simulink model "HAE"  (R2018a)
settings: Solver=ode4  StartTime=0  StopTime=2  MaxStep=1e-4  RelTol=1e-3
InitFcn:
  | close
  | clear
  | clc
  | Sc=128
  | f=60;
  | T=1/f;
  | Ts=1/(f*Sc);
  | Vr=6500
  | V_v=[1    0.4    1          0.6       1       0.6       1       0.75   0.95]
  | T_v=[0   20/f  70/f    200/f   300/f     330/f   400/f   500/f  10]
  | S_time=60/f*20.5
  | V_R=3;
  | Tf=3
  | T_lc=3
  | set_param('HAE/EMISOR-RECEPTOR/TCP_IP_RX1/ESCRITURA', 'Value','0')
  | set_param('HAE/EMISOR-RECEPTOR/TCP_IP_RX1/RETARDO', 'Value','0')
  | run script_client_1_inicio2.m
undefined symbols (not defined in the file or in its folder): D11, Delta, DiscIntNeverNeededParam, Int, Ip1
libraries: powerlib x68, simulink x12, powerlib_meascontrol x6, libreria_comunicaciones_cliente2 x2, libreria_medidores2 x1
(part 4 of 5)

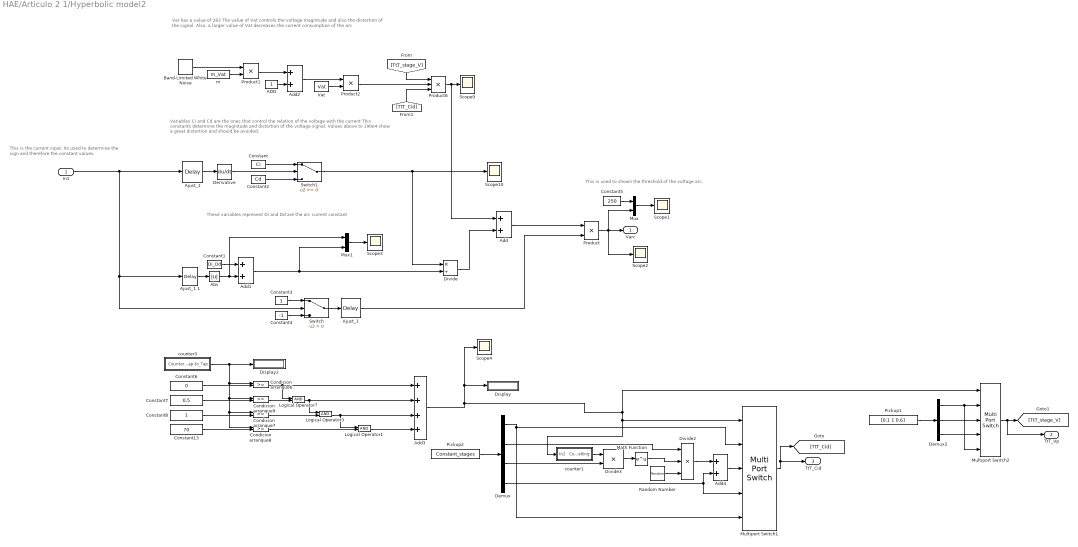
== system HAE/Articulo 2 1/Hyperbolic model2 ==
  note: Vat has a value of 283
      | The value of Vat controls the voltage magnitude and also the distortion of the signal.
      |
      | Also, a larger value of Vat decreases the current consumption of the arc
  note: Variables  Ci and Cd are the ones that control the relation of the voltage with the current
      |
      | This constants determine the magnitude and distortion of the voltage signal.
      |
      | Values above to 190e4 show a great distortion and should be avoided.
  note: These variables represent Di and Dd are the arc current constant
  note: This is used to shown the threshold of the voltage arc.
  note: This is the current input. Its used to determine the sign and therefore the constant values.
  In1 : Inport
  ADD : Constant  SampleTime=Ts
  Abs : Abs
  Add{,1..2,4} (4 alike) : Sum
  Add3 : Sum  Inputs=++++
  Ajust_1 : TransportDelay  DelayTime=1/(1024*60)
  "Ajust_1 " : TransportDelay  DelayTime=1/(1024*60)
  Ajust_1 1 : TransportDelay  DelayTime=1/(1024*60)
  Band-Limited White Noise : simulink/Sources/Band-Limited White Noise  Cov=[0.00005]  Ts=Ts  seed=[500]
  Condicion arranque{6..9} (4 alike) : RelationalOperator  OutDataTypeStr=boolean  RndMeth=Nearest
  Constant : Constant  Value=Ci  SampleTime=Ts
  Constant1 : Constant  Value=Di_Dd  SampleTime=Ts
  Constant13 : Constant  Value=70  VectorParams1D=off  SampleTime=Ts
  Constant2 : Constant  Value=Cd
  Constant3 : Constant
  Constant4 : Constant  Value=-1
  Constant5 : Constant  Value=250
  Constant6 : Constant  Value=0  VectorParams1D=off  SampleTime=Ts
  Constant7 : Constant  Value=0.5  VectorParams1D=off  SampleTime=Ts
  Constant8 : Constant  VectorParams1D=off  SampleTime=Ts
  Demux : Demux
  Demux2 : Demux  Outputs=3
  Derivative : Derivative  CoefficientInTFapproximation=Ts
  Display : Display
  Display2 : Display
  Divide : Product  Inputs=*/
  Divide2 : Product  Inputs=***
  Divide3 : Product  Inputs=**
  Logical Operator1 : Logic  AllPortsSameDT=off  OutDataTypeStr=boolean
  Logical Operator3 : Logic  AllPortsSameDT=off  OutDataTypeStr=boolean
  Logical Operator7 : Logic  AllPortsSameDT=off  OutDataTypeStr=boolean
  Math Function : Math  SaturateOnIntegerOverflow=on
  Multiport Switch1 : MultiPortSwitch  Inputs=4
  Multiport Switch2 : MultiPortSwitch  Inputs=4
  Mux : Mux  Inputs=2
  Mux1 : Mux  Inputs=2
  Pickup1 : Constant  Value=[0.1 1 0.6]
  Pickup2 : Constant  Value=Constant_stages
  Product : Product
  Product1 : Product
  Product2 : Product
  Product6 : Product  Inputs=3
  Random Number : RandomNumber  Mean=2  Variance=0.5  SampleTime=Ts
  Scope{1..4,9..10} (6 alike) : Scope
  Switch : Switch  Criteria=u2 > Threshold  InputSameDT=on
  Switch1 : Switch  InputSameDT=on
  Vat : Constant  Value=Vat  SampleTime=Ts
  counter1 : Subsystem
  counter3 : Subsystem
  "m " : Constant  Value=m_Vat  SampleTime=Ts
  Varc : Outport
  TtT_Vp : Outport  Port=2
  TtT_Cid : Outport  Port=3
  wires:
  Random Number/1 -> Divide2/3
  Add4/1 -> Multiport Switch1/3
  Divide2/1 -> Add4/1
  counter1/1(Counter Melting) -> Divide3/1
  [TtT_Cid] -> Product6/3
  Switch1/1 -> Scope10/1, Divide/1
  Demux2/3 -> Multiport Switch2/4
  Pickup1/1 -> Demux2/1
  Demux2/2 -> Multiport Switch2/3
  Multiport Switch2/1 -> [TtT_stage_V], TtT_Vp/1
  Demux2/1 -> Multiport Switch2/2, Multiport Switch2/5
  Product6/1 -> Scope9/1, Add/1
  Product2/1 -> Product6/2
  [TtT_stage_V] -> Product6/1
  In1/1 -> Ajust_1/1, Ajust_1 1/1, Switch/2
  Add1/1 -> Mux1/2, Divide/2
  Demux/2 -> Divide2/1
  Math Function/1 -> Divide2/2
  Demux/3 -> Divide3/2
  Demux/4 -> Multiport Switch1/4, Add4/2
  Pickup2/1 -> Demux/1
  Divide3/1 -> Math Function/1
  Multiport Switch1/1 -> TtT_Cid/1, [TtT_Cid]
  Demux/1 -> Multiport Switch1/5, Multiport Switch1/2
  Mux1/1 -> Scope3/1
  "Ajust_1 "/1 -> Product/2
  Ajust_1/1 -> Derivative/1
  Derivative/1 -> Switch1/2
  Add2/1 -> Product2/1
  Vat/1 -> Product2/2
  ADD/1 -> Add2/2
  Product1/1 -> Add2/1
  "m "/1 -> Product1/2
  Band-Limited White Noise/1 -> Product1/1
  Abs/1 -> Add1/2, Mux1/1
  Ajust_1 1/1 -> Abs/1
  Constant1/1 -> Add1/1
  Constant5/1 -> Mux/1
  Mux/1 -> Scope1/1
  Constant2/1 -> Switch1/3
  Constant/1 -> Switch1/1
  Product/1 -> Scope2/1, Varc/1, Mux/2
  Switch/1 -> "Ajust_1 "/1
  Constant3/1 -> Switch/1
  Constant4/1 -> Switch/3
  Add/1 -> Product/1
  Divide/1 -> Add/2
  Logical Operator1/1 -> Add3/4
  counter3/1(Counter Tap-to_Tap) -> Condicion arranque9/1, Condicion arranque8/1, Condicion arranque7/1, Condicion arranque6/1, Display2/1
  Condicion arranque7/1 -> Logical Operator3/2
  Logical Operator7/1 -> Add3/2, Logical Operator3/1
  Logical Operator3/1 -> Logical Operator1/1, Add3/3
  Condicion arranque8/1 -> Logical Operator1/2
  Condicion arranque6/1 -> Logical Operator7/1, Add3/1
  Condicion arranque9/1 -> Logical Operator7/2
  Add3/1 -> Multiport Switch2/1, Multiport Switch1/1, counter1/1(In2), Scope4/1, Display/1
  Constant6/1 -> Condicion arranque6/2
  Constant8/1 -> Condicion arranque7/2
  Constant7/1 -> Condicion arranque9/2
  Constant13/1 -> Condicion arranque8/2

== system HAE/Articulo 2 1/counter2 ==
  Add3 : Sum
  Arranq3 : Switch  Threshold=1.5  ZeroCross=off
  Constant1 : Constant  Value=Ts
  Constant3 : Constant  Value=0
  Constant4 : Constant
  Divide : Product  Inputs=**
  Unit Delay1 : UnitDelay  SampleTime=-1
  Unit Delay2 : UnitDelay  SampleTime=-1
  Counter Tap-to_Tap : Outport
  wires:
  Arranq3/1 -> Divide/2
  Add3/1 -> Counter Tap-to_Tap/1, Arranq3/2, Divide/1
  Divide/1 -> Unit Delay1/1
  Constant4/1 -> Arranq3/3
  Constant3/1 -> Arranq3/1
  Unit Delay1/1 -> Add3/2
  Unit Delay2/1 -> Add3/1
  Constant1/1 -> Unit Delay2/1

== system HAE/RB1/RMS1 ==
  In1 : Inport
  Abs : Abs
  Abs1 : Abs
  Abs2 : Abs
  Check zero Crossing : HitCross
  Check zero Crossing1 : HitCross
  Check zero Crossing2 : HitCross
  Constant : Constant  Value=F
  Demux : Demux  Outputs=3
  Discrete Derivative : simulink/Discrete/Discrete Derivative  gainval=1.0  ICPrevScaledInput=0.0  OutMin=[]  OutMax=[]  OutDataType=fixdt(1, 16)  OutScaling=2^-10  DoSatur=off
  Discrete Derivative1 : simulink/Discrete/Discrete Derivative  gainval=1.0  ICPrevScaledInput=0.0  OutMin=[]  OutMax=[]  OutDataType=fixdt(1, 16)  OutScaling=2^-10  DoSatur=off
  Discrete Derivative2 : simulink/Discrete/Discrete Derivative  gainval=1.0  ICPrevScaledInput=0.0  OutMin=[]  OutMax=[]  OutDataType=fixdt(1, 16)  OutScaling=2^-10  DoSatur=off
  Divide : Product  Inputs=/*
  Gain : Gain  Gain=2*pi
  Gain1 : Gain  Gain=1/sqrt(2)
  Hold derivative till next zero crossing : Subsystem  AncestorBlock=|  DialogController=POWERSYS.PowerSysDialog  mask(Discrete Sample & Hold){ic=0, Ts=-1}
      | powerlib_extras/Discrete 
      | Control Blocks/Discrete
      | Sample & Hold
      mask prompts: ic "Initial condition:"; Ts "Sample time:"
      mask help: The output follows input 1 (In) as long as input 2 (S) is TRUE (1) . The output is held when input 2 becomes FALSE (0). The output initial value is specified by the parameter "Initial condition".
      mask init:
      | power_initmask();
      mask Help: This block is part of a subset of blocks in the Extras library that does not have documentation associated with it, other than the block mask description.
      mask Display: disp('S/H')
  Hold derivative till next zero crossing1 : Subsystem  AncestorBlock=|  DialogController=POWERSYS.PowerSysDialog  mask(Discrete Sample & Hold){ic=0, Ts=-1}
      | powerlib_extras/Discrete 
      | Control Blocks/Discrete
      | Sample & Hold
      mask prompts: ic "Initial condition:"; Ts "Sample time:"
      mask help: The output follows input 1 (In) as long as input 2 (S) is TRUE (1) . The output is held when input 2 becomes FALSE (0). The output initial value is specified by the parameter "Initial condition".
      mask init:
      | power_initmask();
      mask Help: This block is part of a subset of blocks in the Extras library that does not have documentation associated with it, other than the block mask description.
      mask Display: disp('S/H')
  Hold derivative till next zero crossing2 : Subsystem  AncestorBlock=|  DialogController=POWERSYS.PowerSysDialog  mask(Discrete Sample & Hold){ic=0, Ts=-1}
      | powerlib_extras/Discrete 
      | Control Blocks/Discrete
      | Sample & Hold
      mask prompts: ic "Initial condition:"; Ts "Sample time:"
      mask help: The output follows input 1 (In) as long as input 2 (S) is TRUE (1) . The output is held when input 2 becomes FALSE (0). The output initial value is specified by the parameter "Initial condition".
      mask init:
      | power_initmask();
      mask Help: This block is part of a subset of blocks in the Extras library that does not have documentation associated with it, other than the block mask description.
      mask Display: disp('S/H')
  Mux : Mux  Inputs=3
  Out1 : Outport
  wires:
  Discrete Derivative/1 -> Hold derivative till next zero crossing/1(In)
  Check zero Crossing/1 -> Hold derivative till next zero crossing/2(S)
  Hold derivative till next zero crossing/1("   ") -> Abs/1
  Constant/1 -> Gain/1
  Gain/1 -> Divide/1
  Abs/1 -> Mux/1
  Demux/1 -> Check zero Crossing/1, Discrete Derivative/1
  Divide/1 -> Gain1/1
  Gain1/1 -> Out1/1
  Hold derivative till next zero crossing1/1("   ") -> Abs1/1
  Check zero Crossing1/1 -> Hold derivative till next zero crossing1/2(S)
  Discrete Derivative1/1 -> Hold derivative till next zero crossing1/1(In)
  Discrete Derivative2/1 -> Hold derivative till next zero crossing2/1(In)
  Check zero Crossing2/1 -> Hold derivative till next zero crossing2/2(S)
  Hold derivative till next zero crossing2/1("   ") -> Abs2/1
  Demux/2 -> Check zero Crossing1/1, Discrete Derivative1/1
  Demux/3 -> Check zero Crossing2/1, Discrete Derivative2/1
  Abs1/1 -> Mux/2
  Mux/1 -> Divide/2
  Abs2/1 -> Mux/3
  In1/1 -> Demux/1

== system HAE/RB1/Timer Proteccion 50 ==
  T.O. : Inport
  Pick-Up : Inport  Port=2
  Entrada : Inport  Port=3
  Arranq3 : Switch  Criteria=u2 ~= 0  Threshold=Ip1
  Arranq6 : Switch  Criteria=u2 ~= 0  Threshold=Ip1  ZeroCross=off
  C14 : Constant  Value=0
  C15 : Constant  Value=1000
  C16 : Constant
  Condicion arranque1 : RelationalOperator  Operator=>  OutDataTypeStr=boolean  RndMeth=Nearest
  Discrete-Time Integrator : DiscreteIntegrator  ExternalReset=falling  SampleTime=-1  ICPrevOutput=DiscIntNeverNeededParam  ICPrevScaledInput=DiscIntNeverNeededParam
  Logical Operator4 : Logic  Operator=NOT  AllPortsSameDT=off  OutDataTypeStr=boolean
  Tiempo Disparo1 : RelationalOperator  OutDataTypeStr=boolean  RndMeth=Nearest
  Trip : Outport
  wires:
  C16/1 -> Arranq6/1
  Arranq6/1 -> Logical Operator4/1, Arranq6/3
  Tiempo Disparo1/1 -> Arranq6/2
  C15/1 -> Arranq3/1
  C14/1 -> Arranq3/3
  Arranq3/1 -> Discrete-Time Integrator/1
  Condicion arranque1/1 -> Arranq3/2, Discrete-Time Integrator/2
  Pick-Up/1 -> Condicion arranque1/2
  Discrete-Time Integrator/1 -> Tiempo Disparo1/1
  Logical Operator4/1 -> Trip/1
  Entrada/1 -> Condicion arranque1/1
  T.O./1 -> Tiempo Disparo1/2

== system HAE/RB1/Timer Proteccion 51 ==
  Entrada : Inport
  Pick-Up : Inport  Port=2
  T.O. : Inport  Port=3
  Arranq3 : Switch  Criteria=u2 ~= 0  Threshold=Ip1
  Arranq6 : Switch  Criteria=u2 ~= 0  Threshold=Ip1  ZeroCross=off
  C14 : Constant  Value=0
  C15 : Constant  Value=1000
  C16 : Constant
  Condicion arranque1 : RelationalOperator  Operator=>  OutDataTypeStr=boolean  RndMeth=Nearest
  Discrete-Time Integrator : DiscreteIntegrator  ExternalReset=falling  SampleTime=-1  ICPrevOutput=DiscIntNeverNeededParam  ICPrevScaledInput=DiscIntNeverNeededParam
  Logical Operator4 : Logic  Operator=NOT  AllPortsSameDT=off  OutDataTypeStr=boolean
  Tiempo Disparo1 : RelationalOperator  OutDataTypeStr=boolean  RndMeth=Nearest
  Trip : Outport
  wires:
  C16/1 -> Arranq6/1
  Arranq6/1 -> Logical Operator4/1, Arranq6/3
  Tiempo Disparo1/1 -> Arranq6/2
  T.O./1 -> Tiempo Disparo1/2
  C15/1 -> Arranq3/1
  C14/1 -> Arranq3/3
  Arranq3/1 -> Discrete-Time Integrator/1
  Condicion arranque1/1 -> Arranq3/2, Discrete-Time Integrator/2
  Pick-Up/1 -> Condicion arranque1/2
  Entrada/1 -> Condicion arranque1/1
  Discrete-Time Integrator/1 -> Tiempo Disparo1/1
  Logical Operator4/1 -> Trip/1

== system HAE/RB4/RMS1 ==
  In1 : Inport
  Abs : Abs
  Abs1 : Abs
  Abs2 : Abs
  Check zero Crossing : HitCross
  Check zero Crossing1 : HitCross
  Check zero Crossing2 : HitCross
  Constant : Constant  Value=F
  Demux : Demux  Outputs=3
  Discrete Derivative : simulink/Discrete/Discrete Derivative  gainval=1.0  ICPrevScaledInput=0.0  OutMin=[]  OutMax=[]  OutDataType=fixdt(1, 16)  OutScaling=2^-10  DoSatur=off
  Discrete Derivative1 : simulink/Discrete/Discrete Derivative  gainval=1.0  ICPrevScaledInput=0.0  OutMin=[]  OutMax=[]  OutDataType=fixdt(1, 16)  OutScaling=2^-10  DoSatur=off
  Discrete Derivative2 : simulink/Discrete/Discrete Derivative  gainval=1.0  ICPrevScaledInput=0.0  OutMin=[]  OutMax=[]  OutDataType=fixdt(1, 16)  OutScaling=2^-10  DoSatur=off
  Divide : Product  Inputs=/*
  Gain : Gain  Gain=2*pi
  Gain1 : Gain  Gain=1/sqrt(2)
  Hold derivative till next zero crossing : Subsystem  AncestorBlock=|  DialogController=POWERSYS.PowerSysDialog  mask(Discrete Sample & Hold){ic=0, Ts=-1}
      | powerlib_extras/Discrete 
      | Control Blocks/Discrete
      | Sample & Hold
      mask prompts: ic "Initial condition:"; Ts "Sample time:"
      mask help: The output follows input 1 (In) as long as input 2 (S) is TRUE (1) . The output is held when input 2 becomes FALSE (0). The output initial value is specified by the parameter "Initial condition".
      mask init:
      | power_initmask();
      mask Help: This block is part of a subset of blocks in the Extras library that does not have documentation associated with it, other than the block mask description.
      mask Display: disp('S/H')
  Hold derivative till next zero crossing1 : Subsystem  AncestorBlock=|  DialogController=POWERSYS.PowerSysDialog  mask(Discrete Sample & Hold){ic=0, Ts=-1}
      | powerlib_extras/Discrete 
      | Control Blocks/Discrete
      | Sample & Hold
      mask prompts: ic "Initial condition:"; Ts "Sample time:"
      mask help: The output follows input 1 (In) as long as input 2 (S) is TRUE (1) . The output is held when input 2 becomes FALSE (0). The output initial value is specified by the parameter "Initial condition".
      mask init:
      | power_initmask();
      mask Help: This block is part of a subset of blocks in the Extras library that does not have documentation associated with it, other than the block mask description.
      mask Display: disp('S/H')
  Hold derivative till next zero crossing2 : Subsystem  AncestorBlock=|  DialogController=POWERSYS.PowerSysDialog  mask(Discrete Sample & Hold){ic=0, Ts=-1}
      | powerlib_extras/Discrete 
      | Control Blocks/Discrete
      | Sample & Hold
      mask prompts: ic "Initial condition:"; Ts "Sample time:"
      mask help: The output follows input 1 (In) as long as input 2 (S) is TRUE (1) . The output is held when input 2 becomes FALSE (0). The output initial value is specified by the parameter "Initial condition".
      mask init:
      | power_initmask();
      mask Help: This block is part of a subset of blocks in the Extras library that does not have documentation associated with it, other than the block mask description.
      mask Display: disp('S/H')
  Mux : Mux  Inputs=3
  Out1 : Outport
  wires:
  In1/1 -> Demux/1
  Abs2/1 -> Mux/3
  Mux/1 -> Divide/2
  Abs1/1 -> Mux/2
  Demux/3 -> Discrete Derivative2/1, Check zero Crossing2/1
  Demux/2 -> Discrete Derivative1/1, Check zero Crossing1/1
  Hold derivative till next zero crossing2/1("   ") -> Abs2/1
  Check zero Crossing2/1 -> Hold derivative till next zero crossing2/2(S)
  Discrete Derivative2/1 -> Hold derivative till next zero crossing2/1(In)
  Discrete Derivative1/1 -> Hold derivative till next zero crossing1/1(In)
  Check zero Crossing1/1 -> Hold derivative till next zero crossing1/2(S)
  Hold derivative till next zero crossing1/1("   ") -> Abs1/1
  Gain1/1 -> Out1/1
  Divide/1 -> Gain1/1
  Demux/1 -> Discrete Derivative/1, Check zero Crossing/1
  Abs/1 -> Mux/1
  Gain/1 -> Divide/1
  Constant/1 -> Gain/1
  Hold derivative till next zero crossing/1("   ") -> Abs/1
  Check zero Crossing/1 -> Hold derivative till next zero crossing/2(S)
  Discrete Derivative/1 -> Hold derivative till next zero crossing/1(In)

== system HAE/RB4/Timer Proteccion 50 ==
  T.O. : Inport
  Pick-Up : Inport  Port=2
  Entrada : Inport  Port=3
  Arranq3 : Switch  Criteria=u2 ~= 0  Threshold=Ip1
  Arranq6 : Switch  Criteria=u2 ~= 0  Threshold=Ip1  ZeroCross=off
  C14 : Constant  Value=0
  C15 : Constant  Value=1000
  C16 : Constant
  Condicion arranque1 : RelationalOperator  Operator=>  OutDataTypeStr=boolean  RndMeth=Nearest
  Discrete-Time Integrator : DiscreteIntegrator  ExternalReset=falling  SampleTime=-1  ICPrevOutput=DiscIntNeverNeededParam  ICPrevScaledInput=DiscIntNeverNeededParam
  Logical Operator4 : Logic  Operator=NOT  AllPortsSameDT=off  OutDataTypeStr=boolean
  Tiempo Disparo1 : RelationalOperator  OutDataTypeStr=boolean  RndMeth=Nearest
  Trip : Outport
  wires:
  T.O./1 -> Tiempo Disparo1/2
  Entrada/1 -> Condicion arranque1/1
  Logical Operator4/1 -> Trip/1
  Discrete-Time Integrator/1 -> Tiempo Disparo1/1
  Pick-Up/1 -> Condicion arranque1/2
  Condicion arranque1/1 -> Discrete-Time Integrator/2, Arranq3/2
  Arranq3/1 -> Discrete-Time Integrator/1
  C14/1 -> Arranq3/3
  C15/1 -> Arranq3/1
  Tiempo Disparo1/1 -> Arranq6/2
  Arranq6/1 -> Arranq6/3, Logical Operator4/1
  C16/1 -> Arranq6/1

== system HAE/RB4/Timer Proteccion 51 ==
  Entrada : Inport
  Pick-Up : Inport  Port=2
  T.O. : Inport  Port=3
  Arranq3 : Switch  Criteria=u2 ~= 0  Threshold=Ip1
  Arranq6 : Switch  Criteria=u2 ~= 0  Threshold=Ip1  ZeroCross=off
  C14 : Constant  Value=0
  C15 : Constant  Value=1000
  C16 : Constant
  Condicion arranque1 : RelationalOperator  Operator=>  OutDataTypeStr=boolean  RndMeth=Nearest
  Discrete-Time Integrator : DiscreteIntegrator  ExternalReset=falling  SampleTime=-1  ICPrevOutput=DiscIntNeverNeededParam  ICPrevScaledInput=DiscIntNeverNeededParam
  Logical Operator4 : Logic  Operator=NOT  AllPortsSameDT=off  OutDataTypeStr=boolean
  Tiempo Disparo1 : RelationalOperator  OutDataTypeStr=boolean  RndMeth=Nearest
  Trip : Outport
  wires:
  Logical Operator4/1 -> Trip/1
  Discrete-Time Integrator/1 -> Tiempo Disparo1/1
  Entrada/1 -> Condicion arranque1/1
  Pick-Up/1 -> Condicion arranque1/2
  Condicion arranque1/1 -> Discrete-Time Integrator/2, Arranq3/2
  Arranq3/1 -> Discrete-Time Integrator/1
  C14/1 -> Arranq3/3
  C15/1 -> Arranq3/1
  T.O./1 -> Tiempo Disparo1/2
  Tiempo Disparo1/1 -> Arranq6/2
  Arranq6/1 -> Arranq6/3, Logical Operator4/1
  C16/1 -> Arranq6/1

== system HAE/RB5/RMS1 ==
  In1 : Inport
  Abs : Abs
  Abs1 : Abs
  Abs2 : Abs
  Check zero Crossing : HitCross
  Check zero Crossing1 : HitCross
  Check zero Crossing2 : HitCross
  Constant : Constant  Value=F
  Demux : Demux  Outputs=3
  Discrete Derivative : simulink/Discrete/Discrete Derivative  gainval=1.0  ICPrevScaledInput=0.0  OutMin=[]  OutMax=[]  OutDataType=fixdt(1, 16)  OutScaling=2^-10  DoSatur=off
  Discrete Derivative1 : simulink/Discrete/Discrete Derivative  gainval=1.0  ICPrevScaledInput=0.0  OutMin=[]  OutMax=[]  OutDataType=fixdt(1, 16)  OutScaling=2^-10  DoSatur=off
  Discrete Derivative2 : simulink/Discrete/Discrete Derivative  gainval=1.0  ICPrevScaledInput=0.0  OutMin=[]  OutMax=[]  OutDataType=fixdt(1, 16)  OutScaling=2^-10  DoSatur=off
  Divide : Product  Inputs=/*
  Gain : Gain  Gain=2*pi
  Gain1 : Gain  Gain=1/sqrt(2)
  Hold derivative till next zero crossing : Subsystem  AncestorBlock=|  DialogController=POWERSYS.PowerSysDialog  mask(Discrete Sample & Hold){ic=0, Ts=-1}
      | powerlib_extras/Discrete 
      | Control Blocks/Discrete
      | Sample & Hold
      mask prompts: ic "Initial condition:"; Ts "Sample time:"
      mask help: The output follows input 1 (In) as long as input 2 (S) is TRUE (1) . The output is held when input 2 becomes FALSE (0). The output initial value is specified by the parameter "Initial condition".
      mask init:
      | power_initmask();
      mask Help: This block is part of a subset of blocks in the Extras library that does not have documentation associated with it, other than the block mask description.
      mask Display: disp('S/H')
  Hold derivative till next zero crossing1 : Subsystem  AncestorBlock=|  DialogController=POWERSYS.PowerSysDialog  mask(Discrete Sample & Hold){ic=0, Ts=-1}
      | powerlib_extras/Discrete 
      | Control Blocks/Discrete
      | Sample & Hold
      mask prompts: ic "Initial condition:"; Ts "Sample time:"
      mask help: The output follows input 1 (In) as long as input 2 (S) is TRUE (1) . The output is held when input 2 becomes FALSE (0). The output initial value is specified by the parameter "Initial condition".
      mask init:
      | power_initmask();
      mask Help: This block is part of a subset of blocks in the Extras library that does not have documentation associated with it, other than the block mask description.
      mask Display: disp('S/H')
  Hold derivative till next zero crossing2 : Subsystem  AncestorBlock=|  DialogController=POWERSYS.PowerSysDialog  mask(Discrete Sample & Hold){ic=0, Ts=-1}
      | powerlib_extras/Discrete 
      | Control Blocks/Discrete
      | Sample & Hold
      mask prompts: ic "Initial condition:"; Ts "Sample time:"
      mask help: The output follows input 1 (In) as long as input 2 (S) is TRUE (1) . The output is held when input 2 becomes FALSE (0). The output initial value is specified by the parameter "Initial condition".
      mask init:
      | power_initmask();
      mask Help: This block is part of a subset of blocks in the Extras library that does not have documentation associated with it, other than the block mask description.
      mask Display: disp('S/H')
  Mux : Mux  Inputs=3
  Out1 : Outport
  wires:
  Discrete Derivative/1 -> Hold derivative till next zero crossing/1(In)
  Check zero Crossing/1 -> Hold derivative till next zero crossing/2(S)
  Hold derivative till next zero crossing/1("   ") -> Abs/1
  Constant/1 -> Gain/1
  Gain/1 -> Divide/1
  Abs/1 -> Mux/1
  Demux/1 -> Check zero Crossing/1, Discrete Derivative/1
  Divide/1 -> Gain1/1
  Gain1/1 -> Out1/1
  Hold derivative till next zero crossing1/1("   ") -> Abs1/1
  Check zero Crossing1/1 -> Hold derivative till next zero crossing1/2(S)
  Discrete Derivative1/1 -> Hold derivative till next zero crossing1/1(In)
  Discrete Derivative2/1 -> Hold derivative till next zero crossing2/1(In)
  Check zero Crossing2/1 -> Hold derivative till next zero crossing2/2(S)
  Hold derivative till next zero crossing2/1("   ") -> Abs2/1
  Demux/2 -> Check zero Crossing1/1, Discrete Derivative1/1
  Demux/3 -> Check zero Crossing2/1, Discrete Derivative2/1
  Abs1/1 -> Mux/2
  Mux/1 -> Divide/2
  Abs2/1 -> Mux/3
  In1/1 -> Demux/1

== system HAE/RB5/Timer Proteccion 50 ==
  T.O. : Inport
  Pick-Up : Inport  Port=2
  Entrada : Inport  Port=3
  Arranq3 : Switch  Criteria=u2 ~= 0  Threshold=Ip1
  Arranq6 : Switch  Criteria=u2 ~= 0  Threshold=Ip1  ZeroCross=off
  C14 : Constant  Value=0
  C15 : Constant  Value=1000
  C16 : Constant
  Condicion arranque1 : RelationalOperator  Operator=>  OutDataTypeStr=boolean  RndMeth=Nearest
  Discrete-Time Integrator : DiscreteIntegrator  ExternalReset=falling  SampleTime=-1  ICPrevOutput=DiscIntNeverNeededParam  ICPrevScaledInput=DiscIntNeverNeededParam
  Logical Operator4 : Logic  Operator=NOT  AllPortsSameDT=off  OutDataTypeStr=boolean
  Tiempo Disparo1 : RelationalOperator  OutDataTypeStr=boolean  RndMeth=Nearest
  Trip : Outport
  wires:
  C16/1 -> Arranq6/1
  Arranq6/1 -> Logical Operator4/1, Arranq6/3
  Tiempo Disparo1/1 -> Arranq6/2
  C15/1 -> Arranq3/1
  C14/1 -> Arranq3/3
  Arranq3/1 -> Discrete-Time Integrator/1
  Condicion arranque1/1 -> Arranq3/2, Discrete-Time Integrator/2
  Pick-Up/1 -> Condicion arranque1/2
  Discrete-Time Integrator/1 -> Tiempo Disparo1/1
  Logical Operator4/1 -> Trip/1
  Entrada/1 -> Condicion arranque1/1
  T.O./1 -> Tiempo Disparo1/2

== system HAE/RB5/Timer Proteccion 51 ==
  Entrada : Inport
  Pick-Up : Inport  Port=2
  T.O. : Inport  Port=3
  Arranq3 : Switch  Criteria=u2 ~= 0  Threshold=Ip1
  Arranq6 : Switch  Criteria=u2 ~= 0  Threshold=Ip1  ZeroCross=off
  C14 : Constant  Value=0
  C15 : Constant  Value=1000
  C16 : Constant
  Condicion arranque1 : RelationalOperator  Operator=>  OutDataTypeStr=boolean  RndMeth=Nearest
  Discrete-Time Integrator : DiscreteIntegrator  ExternalReset=falling  SampleTime=-1  ICPrevOutput=DiscIntNeverNeededParam  ICPrevScaledInput=DiscIntNeverNeededParam
  Logical Operator4 : Logic  Operator=NOT  AllPortsSameDT=off  OutDataTypeStr=boolean
  Tiempo Disparo1 : RelationalOperator  OutDataTypeStr=boolean  RndMeth=Nearest
  Trip : Outport
  wires:
  C16/1 -> Arranq6/1
  Arranq6/1 -> Logical Operator4/1, Arranq6/3
  Tiempo Disparo1/1 -> Arranq6/2
  T.O./1 -> Tiempo Disparo1/2
  C15/1 -> Arranq3/1
  C14/1 -> Arranq3/3
  Arranq3/1 -> Discrete-Time Integrator/1
  Condicion arranque1/1 -> Arranq3/2, Discrete-Time Integrator/2
  Pick-Up/1 -> Condicion arranque1/2
  Entrada/1 -> Condicion arranque1/1
  Discrete-Time Integrator/1 -> Tiempo Disparo1/1
  Logical Operator4/1 -> Trip/1

== system HAE/Subsystem1/RMS ==
  In1 : Inport
  Absolute : MATLABFcn  MATLABFcn=abs
  Check zero Crossing : HitCross
  Constant : Constant  Value=F
  Derivative : Derivative
  Divide : Product  Inputs=/*
  Gain : Gain  Gain=2*pi
  Gain1 : Gain  Gain=1/sqrt(2)
  Hold derivative till next zero crossing : Subsystem  AncestorBlock=|  DialogController=POWERSYS.PowerSysDialog  mask(Discrete Sample & Hold){ic=0, Ts=-1}
      | powerlib_extras/Discrete 
      | Control Blocks/Discrete
      | Sample & Hold
      mask prompts: ic "Initial condition:"; Ts "Sample time:"
      mask help: The output follows input 1 (In) as long as input 2 (S) is TRUE (1) . The output is held when input 2 becomes FALSE (0). The output initial value is specified by the parameter "Initial condition".
      mask init:
      | power_initmask();
      mask Help: This block is part of a subset of blocks in the Extras library that does not have documentation associated with it, other than the block mask description.
      mask Display: disp('S/H')
  Out1 : Outport
  wires:
  Derivative/1 -> Hold derivative till next zero crossing/1(In)
  Check zero Crossing/1 -> Hold derivative till next zero crossing/2(S)
  Hold derivative till next zero crossing/1("   ") -> Absolute/1
  Constant/1 -> Gain/1
  Gain/1 -> Divide/1
  Absolute/1 -> Divide/2
  In1/1 -> Check zero Crossing/1, Derivative/1
  Divide/1 -> Gain1/1
  Gain1/1 -> Out1/1

== system HAE/Subsystem1/Timer Proteccion ==
  Entrada : Inport
  Pick-Up : Inport  Port=2
  T.O. : Inport  Port=3
  Arranq3 : Switch  Criteria=u2 ~= 0  Threshold=Ip1
  Arranq6 : Switch  Criteria=u2 ~= 0  Threshold=Ip1  ZeroCross=off
  C14 : Constant  Value=0
  C15 : Constant  Value=1000
  C16 : Constant
  Condicion arranque1 : RelationalOperator  Operator=>  OutDataTypeStr=boolean  RndMeth=Nearest
  Discrete-Time Integrator : DiscreteIntegrator  ExternalReset=falling  SampleTime=-1  ICPrevOutput=DiscIntNeverNeededParam  ICPrevScaledInput=DiscIntNeverNeededParam
  Logical Operator4 : Logic  Operator=NOT  AllPortsSameDT=off  OutDataTypeStr=boolean
  Tiempo Disparo1 : RelationalOperator  Operator=>  OutDataTypeStr=boolean  RndMeth=Nearest
  Trip : Outport
  wires:
  C16/1 -> Arranq6/1
  Arranq6/1 -> Logical Operator4/1, Arranq6/3
  Tiempo Disparo1/1 -> Arranq6/2
  T.O./1 -> Tiempo Disparo1/2
  C15/1 -> Arranq3/1
  C14/1 -> Arranq3/3
  Arranq3/1 -> Discrete-Time Integrator/1
  Condicion arranque1/1 -> Arranq3/2, Discrete-Time Integrator/2
  Pick-Up/1 -> Condicion arranque1/2
  Entrada/1 -> Condicion arranque1/1
  Discrete-Time Integrator/1 -> Tiempo Disparo1/1
  Logical Operator4/1 -> Trip/1

== system HAE/Subsystem1/Timer Proteccion1 ==
  Entrada : Inport
  Pick-Up : Inport  Port=2
  T.O. : Inport  Port=3
  Arranq3 : Switch  Criteria=u2 ~= 0  Threshold=Ip1
  Arranq6 : Switch  Criteria=u2 ~= 0  Threshold=Ip1  ZeroCross=off
  C14 : Constant  Value=0
  C15 : Constant  Value=1000
  C16 : Constant
  Condicion arranque1 : RelationalOperator  Operator=>  OutDataTypeStr=boolean  RndMeth=Nearest
  Discrete-Time Integrator : DiscreteIntegrator  ExternalReset=falling  SampleTime=-1  ICPrevOutput=DiscIntNeverNeededParam  ICPrevScaledInput=DiscIntNeverNeededParam
  Logical Operator4 : Logic  Operator=NOT  AllPortsSameDT=off  OutDataTypeStr=boolean
  Scope1 : Scope  NumInputPorts=2
  Tiempo Disparo1 : RelationalOperator  Operator=>  OutDataTypeStr=boolean  RndMeth=Nearest
  Trip : Outport
  wires:
  C16/1 -> Arranq6/1
  Arranq6/1 -> Logical Operator4/1, Arranq6/3
  Tiempo Disparo1/1 -> Arranq6/2
  T.O./1 -> Tiempo Disparo1/2
  C15/1 -> Arranq3/1
  C14/1 -> Arranq3/3
  Arranq3/1 -> Discrete-Time Integrator/1
  Condicion arranque1/1 -> Scope1/1, Arranq3/2, Discrete-Time Integrator/2
  Pick-Up/1 -> Condicion arranque1/2
  Entrada/1 -> Condicion arranque1/1
  Discrete-Time Integrator/1 -> Scope1/2, Tiempo Disparo1/1
  Logical Operator4/1 -> Trip/1

== system HAE/Subsystem10/RMS ==
  In1 : Inport
  Absolute : MATLABFcn  MATLABFcn=abs
  Check zero Crossing : HitCross
  Constant : Constant  Value=F
  Derivative : Derivative
  Divide : Product  Inputs=/*
  Gain : Gain  Gain=2*pi
  Gain1 : Gain  Gain=1/sqrt(2)
  Hold derivative till next zero crossing : Subsystem  AncestorBlock=|  DialogController=POWERSYS.PowerSysDialog  mask(Discrete Sample & Hold){ic=0, Ts=-1}
      | powerlib_extras/Discrete 
      | Control Blocks/Discrete
      | Sample & Hold
      mask prompts: ic "Initial condition:"; Ts "Sample time:"
      mask help: The output follows input 1 (In) as long as input 2 (S) is TRUE (1) . The output is held when input 2 becomes FALSE (0). The output initial value is specified by the parameter "Initial condition".
      mask init:
      | power_initmask();
      mask Help: This block is part of a subset of blocks in the Extras library that does not have documentation associated with it, other than the block mask description.
      mask Display: disp('S/H')
  Out1 : Outport
  wires:
  Derivative/1 -> Hold derivative till next zero crossing/1(In)
  Check zero Crossing/1 -> Hold derivative till next zero crossing/2(S)
  Hold derivative till next zero crossing/1("   ") -> Absolute/1
  Constant/1 -> Gain/1
  Gain/1 -> Divide/1
  Absolute/1 -> Divide/2
  In1/1 -> Check zero Crossing/1, Derivative/1
  Divide/1 -> Gain1/1
  Gain1/1 -> Out1/1

== system HAE/Subsystem10/Timer Proteccion ==
  Entrada : Inport
  Pick-Up : Inport  Port=2
  T.O. : Inport  Port=3
  Arranq3 : Switch  Criteria=u2 ~= 0  Threshold=Ip1
  Arranq6 : Switch  Criteria=u2 ~= 0  Threshold=Ip1  ZeroCross=off
  C14 : Constant  Value=0
  C15 : Constant  Value=1000
  C16 : Constant
  Condicion arranque1 : RelationalOperator  Operator=>  OutDataTypeStr=boolean  RndMeth=Nearest
  Discrete-Time Integrator : DiscreteIntegrator  ExternalReset=falling  SampleTime=-1  ICPrevOutput=DiscIntNeverNeededParam  ICPrevScaledInput=DiscIntNeverNeededParam
  Logical Operator4 : Logic  Operator=NOT  AllPortsSameDT=off  OutDataTypeStr=boolean
  Tiempo Disparo1 : RelationalOperator  Operator=>  OutDataTypeStr=boolean  RndMeth=Nearest
  Trip : Outport
  wires:
  C16/1 -> Arranq6/1
  Arranq6/1 -> Logical Operator4/1, Arranq6/3
  Tiempo Disparo1/1 -> Arranq6/2
  T.O./1 -> Tiempo Disparo1/2
  C15/1 -> Arranq3/1
  C14/1 -> Arranq3/3
  Arranq3/1 -> Discrete-Time Integrator/1
  Condicion arranque1/1 -> Arranq3/2, Discrete-Time Integrator/2
  Pick-Up/1 -> Condicion arranque1/2
  Entrada/1 -> Condicion arranque1/1
  Discrete-Time Integrator/1 -> Tiempo Disparo1/1
  Logical Operator4/1 -> Trip/1

== system HAE/Subsystem10/Timer Proteccion1 ==
  Entrada : Inport
  Pick-Up : Inport  Port=2
  T.O. : Inport  Port=3
  Arranq3 : Switch  Criteria=u2 ~= 0  Threshold=Ip1
  Arranq6 : Switch  Criteria=u2 ~= 0  Threshold=Ip1  ZeroCross=off
  C14 : Constant  Value=0
  C15 : Constant  Value=1000
  C16 : Constant
  Condicion arranque1 : RelationalOperator  Operator=>  OutDataTypeStr=boolean  RndMeth=Nearest
  Discrete-Time Integrator : DiscreteIntegrator  ExternalReset=falling  SampleTime=-1  ICPrevOutput=DiscIntNeverNeededParam  ICPrevScaledInput=DiscIntNeverNeededParam
  Logical Operator4 : Logic  Operator=NOT  AllPortsSameDT=off  OutDataTypeStr=boolean
  Scope1 : Scope  NumInputPorts=2
  Tiempo Disparo1 : RelationalOperator  Operator=>  OutDataTypeStr=boolean  RndMeth=Nearest
  Trip : Outport
  wires:
  C16/1 -> Arranq6/1
  Arranq6/1 -> Logical Operator4/1, Arranq6/3
  Tiempo Disparo1/1 -> Arranq6/2
  T.O./1 -> Tiempo Disparo1/2
  C15/1 -> Arranq3/1
  C14/1 -> Arranq3/3
  Arranq3/1 -> Discrete-Time Integrator/1
  Condicion arranque1/1 -> Scope1/1, Arranq3/2, Discrete-Time Integrator/2
  Pick-Up/1 -> Condicion arranque1/2
  Entrada/1 -> Condicion arranque1/1
  Discrete-Time Integrator/1 -> Scope1/2, Tiempo Disparo1/1
  Logical Operator4/1 -> Trip/1

== system HAE/Subsystem3/RMS ==
  In1 : Inport
  Absolute : MATLABFcn  MATLABFcn=abs
  Check zero Crossing : HitCross
  Constant : Constant  Value=F
  Derivative : Derivative
  Divide : Product  Inputs=/*
  Gain : Gain  Gain=2*pi
  Gain1 : Gain  Gain=1/sqrt(2)
  Hold derivative till next zero crossing : Subsystem  AncestorBlock=|  DialogController=POWERSYS.PowerSysDialog  mask(Discrete Sample & Hold){ic=0, Ts=-1}
      | powerlib_extras/Discrete 
      | Control Blocks/Discrete
      | Sample & Hold
      mask prompts: ic "Initial condition:"; Ts "Sample time:"
      mask help: The output follows input 1 (In) as long as input 2 (S) is TRUE (1) . The output is held when input 2 becomes FALSE (0). The output initial value is specified by the parameter "Initial condition".
      mask init:
      | power_initmask();
      mask Help: This block is part of a subset of blocks in the Extras library that does not have documentation associated with it, other than the block mask description.
      mask Display: disp('S/H')
  Out1 : Outport
  wires:
  Derivative/1 -> Hold derivative till next zero crossing/1(In)
  Check zero Crossing/1 -> Hold derivative till next zero crossing/2(S)
  Hold derivative till next zero crossing/1("   ") -> Absolute/1
  Constant/1 -> Gain/1
  Gain/1 -> Divide/1
  Absolute/1 -> Divide/2
  In1/1 -> Check zero Crossing/1, Derivative/1
  Divide/1 -> Gain1/1
  Gain1/1 -> Out1/1

== system HAE/Subsystem3/Timer Proteccion ==
  Entrada : Inport
  Pick-Up : Inport  Port=2
  T.O. : Inport  Port=3
  Arranq3 : Switch  Criteria=u2 ~= 0  Threshold=Ip1
  Arranq6 : Switch  Criteria=u2 ~= 0  Threshold=Ip1  ZeroCross=off
  C14 : Constant  Value=0
  C15 : Constant  Value=1000
  C16 : Constant
  Condicion arranque1 : RelationalOperator  Operator=>  OutDataTypeStr=boolean  RndMeth=Nearest
  Discrete-Time Integrator : DiscreteIntegrator  ExternalReset=falling  SampleTime=-1  ICPrevOutput=DiscIntNeverNeededParam  ICPrevScaledInput=DiscIntNeverNeededParam
  Logical Operator4 : Logic  Operator=NOT  AllPortsSameDT=off  OutDataTypeStr=boolean
  Tiempo Disparo1 : RelationalOperator  Operator=>  OutDataTypeStr=boolean  RndMeth=Nearest
  Trip : Outport
  wires:
  C16/1 -> Arranq6/1
  Arranq6/1 -> Logical Operator4/1, Arranq6/3
  Tiempo Disparo1/1 -> Arranq6/2
  T.O./1 -> Tiempo Disparo1/2
  C15/1 -> Arranq3/1
  C14/1 -> Arranq3/3
  Arranq3/1 -> Discrete-Time Integrator/1
  Condicion arranque1/1 -> Arranq3/2, Discrete-Time Integrator/2
  Pick-Up/1 -> Condicion arranque1/2
  Entrada/1 -> Condicion arranque1/1
  Discrete-Time Integrator/1 -> Tiempo Disparo1/1
  Logical Operator4/1 -> Trip/1

== system HAE/Subsystem3/Timer Proteccion1 ==
  Entrada : Inport
  Pick-Up : Inport  Port=2
  T.O. : Inport  Port=3
  Arranq3 : Switch  Criteria=u2 ~= 0  Threshold=Ip1
  Arranq6 : Switch  Criteria=u2 ~= 0  Threshold=Ip1  ZeroCross=off
  C14 : Constant  Value=0
  C15 : Constant  Value=1000
  C16 : Constant
  Condicion arranque1 : RelationalOperator  Operator=>  OutDataTypeStr=boolean  RndMeth=Nearest
  Discrete-Time Integrator : DiscreteIntegrator  ExternalReset=falling  SampleTime=-1  ICPrevOutput=DiscIntNeverNeededParam  ICPrevScaledInput=DiscIntNeverNeededParam
  Logical Operator4 : Logic  Operator=NOT  AllPortsSameDT=off  OutDataTypeStr=boolean
  Scope1 : Scope  NumInputPorts=2
  Tiempo Disparo1 : RelationalOperator  Operator=>  OutDataTypeStr=boolean  RndMeth=Nearest
  Trip : Outport
  wires:
  C16/1 -> Arranq6/1
  Arranq6/1 -> Logical Operator4/1, Arranq6/3
  Tiempo Disparo1/1 -> Arranq6/2
  T.O./1 -> Tiempo Disparo1/2
  C15/1 -> Arranq3/1
  C14/1 -> Arranq3/3
  Arranq3/1 -> Discrete-Time Integrator/1
  Condicion arranque1/1 -> Scope1/1, Arranq3/2, Discrete-Time Integrator/2
  Pick-Up/1 -> Condicion arranque1/2
  Entrada/1 -> Condicion arranque1/1
  Discrete-Time Integrator/1 -> Scope1/2, Tiempo Disparo1/1
  Logical Operator4/1 -> Trip/1

== system HAE/Subsystem6/RMS ==
  In1 : Inport
  Absolute : MATLABFcn  MATLABFcn=abs
  Check zero Crossing : HitCross
  Constant : Constant  Value=F
  Derivative : Derivative
  Divide : Product  Inputs=/*
  Gain : Gain  Gain=2*pi
  Gain1 : Gain  Gain=1/sqrt(2)
  Hold derivative till next zero crossing : Subsystem  AncestorBlock=|  DialogController=POWERSYS.PowerSysDialog  mask(Discrete Sample & Hold){ic=0, Ts=-1}
      | powerlib_extras/Discrete 
      | Control Blocks/Discrete
      | Sample & Hold
      mask prompts: ic "Initial condition:"; Ts "Sample time:"
      mask help: The output follows input 1 (In) as long as input 2 (S) is TRUE (1) . The output is held when input 2 becomes FALSE (0). The output initial value is specified by the parameter "Initial condition".
      mask init:
      | power_initmask();
      mask Help: This block is part of a subset of blocks in the Extras library that does not have documentation associated with it, other than the block mask description.
      mask Display: disp('S/H')
  Out1 : Outport
  wires:
  Derivative/1 -> Hold derivative till next zero crossing/1(In)
  Check zero Crossing/1 -> Hold derivative till next zero crossing/2(S)
  Hold derivative till next zero crossing/1("   ") -> Absolute/1
  Constant/1 -> Gain/1
  Gain/1 -> Divide/1
  Absolute/1 -> Divide/2
  In1/1 -> Check zero Crossing/1, Derivative/1
  Divide/1 -> Gain1/1
  Gain1/1 -> Out1/1

== system HAE/Subsystem6/Timer Proteccion ==
  Entrada : Inport
  Pick-Up : Inport  Port=2
  T.O. : Inport  Port=3
  Arranq3 : Switch  Criteria=u2 ~= 0  Threshold=Ip1
  Arranq6 : Switch  Criteria=u2 ~= 0  Threshold=Ip1  ZeroCross=off
  C14 : Constant  Value=0
  C15 : Constant  Value=1000
  C16 : Constant
  Condicion arranque1 : RelationalOperator  Operator=>  OutDataTypeStr=boolean  RndMeth=Nearest
  Discrete-Time Integrator : DiscreteIntegrator  ExternalReset=falling  SampleTime=-1  ICPrevOutput=DiscIntNeverNeededParam  ICPrevScaledInput=DiscIntNeverNeededParam
  Logical Operator4 : Logic  Operator=NOT  AllPortsSameDT=off  OutDataTypeStr=boolean
  Tiempo Disparo1 : RelationalOperator  Operator=>  OutDataTypeStr=boolean  RndMeth=Nearest
  Trip : Outport
  wires:
  C16/1 -> Arranq6/1
  Arranq6/1 -> Logical Operator4/1, Arranq6/3
  Tiempo Disparo1/1 -> Arranq6/2
  T.O./1 -> Tiempo Disparo1/2
  C15/1 -> Arranq3/1
  C14/1 -> Arranq3/3
  Arranq3/1 -> Discrete-Time Integrator/1
  Condicion arranque1/1 -> Arranq3/2, Discrete-Time Integrator/2
  Pick-Up/1 -> Condicion arranque1/2
  Entrada/1 -> Condicion arranque1/1
  Discrete-Time Integrator/1 -> Tiempo Disparo1/1
  Logical Operator4/1 -> Trip/1

== system HAE/Subsystem6/Timer Proteccion1 ==
  Entrada : Inport
  Pick-Up : Inport  Port=2
  T.O. : Inport  Port=3
  Arranq3 : Switch  Criteria=u2 ~= 0  Threshold=Ip1
  Arranq6 : Switch  Criteria=u2 ~= 0  Threshold=Ip1  ZeroCross=off
  C14 : Constant  Value=0
  C15 : Constant  Value=1000
  C16 : Constant
  Condicion arranque1 : RelationalOperator  Operator=>  OutDataTypeStr=boolean  RndMeth=Nearest
  Discrete-Time Integrator : DiscreteIntegrator  ExternalReset=falling  SampleTime=-1  ICPrevOutput=DiscIntNeverNeededParam  ICPrevScaledInput=DiscIntNeverNeededParam
  Logical Operator4 : Logic  Operator=NOT  AllPortsSameDT=off  OutDataTypeStr=boolean
  Scope1 : Scope  NumInputPorts=2
  Tiempo Disparo1 : RelationalOperator  Operator=>  OutDataTypeStr=boolean  RndMeth=Nearest
  Trip : Outport
  wires:
  C16/1 -> Arranq6/1
  Arranq6/1 -> Logical Operator4/1, Arranq6/3
  Tiempo Disparo1/1 -> Arranq6/2
  T.O./1 -> Tiempo Disparo1/2
  C15/1 -> Arranq3/1
  C14/1 -> Arranq3/3
  Arranq3/1 -> Discrete-Time Integrator/1
  Condicion arranque1/1 -> Scope1/1, Arranq3/2, Discrete-Time Integrator/2
  Pick-Up/1 -> Condicion arranque1/2
  Entrada/1 -> Condicion arranque1/1
  Discrete-Time Integrator/1 -> Scope1/2, Tiempo Disparo1/1
  Logical Operator4/1 -> Trip/1

== system HAE/Subsystem7/RMS ==
  In1 : Inport
  Absolute : MATLABFcn  MATLABFcn=abs
  Check zero Crossing : HitCross
  Constant : Constant  Value=F
  Derivative : Derivative
  Divide : Product  Inputs=/*
  Gain : Gain  Gain=2*pi
  Gain1 : Gain  Gain=1/sqrt(2)
  Hold derivative till next zero crossing : Subsystem  AncestorBlock=|  DialogController=POWERSYS.PowerSysDialog  mask(Discrete Sample & Hold){ic=0, Ts=-1}
      | powerlib_extras/Discrete 
      | Control Blocks/Discrete
      | Sample & Hold
      mask prompts: ic "Initial condition:"; Ts "Sample time:"
      mask help: The output follows input 1 (In) as long as input 2 (S) is TRUE (1) . The output is held when input 2 becomes FALSE (0). The output initial value is specified by the parameter "Initial condition".
      mask init:
      | power_initmask();
      mask Help: This block is part of a subset of blocks in the Extras library that does not have documentation associated with it, other than the block mask description.
      mask Display: disp('S/H')
  Out1 : Outport
  wires:
  Derivative/1 -> Hold derivative till next zero crossing/1(In)
  Check zero Crossing/1 -> Hold derivative till next zero crossing/2(S)
  Hold derivative till next zero crossing/1("   ") -> Absolute/1
  Constant/1 -> Gain/1
  Gain/1 -> Divide/1
  Absolute/1 -> Divide/2
  In1/1 -> Check zero Crossing/1, Derivative/1
  Divide/1 -> Gain1/1
  Gain1/1 -> Out1/1

== system HAE/Subsystem7/Timer Proteccion ==
  Entrada : Inport
  Pick-Up : Inport  Port=2
  T.O. : Inport  Port=3
  Arranq3 : Switch  Criteria=u2 ~= 0  Threshold=Ip1
  Arranq6 : Switch  Criteria=u2 ~= 0  Threshold=Ip1  ZeroCross=off
  C14 : Constant  Value=0
  C15 : Constant  Value=1000
  C16 : Constant
  Condicion arranque1 : RelationalOperator  Operator=>  OutDataTypeStr=boolean  RndMeth=Nearest
  Discrete-Time Integrator : DiscreteIntegrator  ExternalReset=falling  SampleTime=-1  ICPrevOutput=DiscIntNeverNeededParam  ICPrevScaledInput=DiscIntNeverNeededParam
  Logical Operator4 : Logic  Operator=NOT  AllPortsSameDT=off  OutDataTypeStr=boolean
  Tiempo Disparo1 : RelationalOperator  Operator=>  OutDataTypeStr=boolean  RndMeth=Nearest
  Trip : Outport
  wires:
  C16/1 -> Arranq6/1
  Arranq6/1 -> Logical Operator4/1, Arranq6/3
  Tiempo Disparo1/1 -> Arranq6/2
  T.O./1 -> Tiempo Disparo1/2
  C15/1 -> Arranq3/1
  C14/1 -> Arranq3/3
  Arranq3/1 -> Discrete-Time Integrator/1
  Condicion arranque1/1 -> Arranq3/2, Discrete-Time Integrator/2
  Pick-Up/1 -> Condicion arranque1/2
  Entrada/1 -> Condicion arranque1/1
  Discrete-Time Integrator/1 -> Tiempo Disparo1/1
  Logical Operator4/1 -> Trip/1

== system HAE/Subsystem7/Timer Proteccion1 ==
  Entrada : Inport
  Pick-Up : Inport  Port=2
  T.O. : Inport  Port=3
  Arranq3 : Switch  Criteria=u2 ~= 0  Threshold=Ip1
  Arranq6 : Switch  Criteria=u2 ~= 0  Threshold=Ip1  ZeroCross=off
  C14 : Constant  Value=0
  C15 : Constant  Value=1000
  C16 : Constant
  Condicion arranque1 : RelationalOperator  Operator=>  OutDataTypeStr=boolean  RndMeth=Nearest
  Discrete-Time Integrator : DiscreteIntegrator  ExternalReset=falling  SampleTime=-1  ICPrevOutput=DiscIntNeverNeededParam  ICPrevScaledInput=DiscIntNeverNeededParam
  Logical Operator4 : Logic  Operator=NOT  AllPortsSameDT=off  OutDataTypeStr=boolean
  Scope1 : Scope  NumInputPorts=2
  Tiempo Disparo1 : RelationalOperator  Operator=>  OutDataTypeStr=boolean  RndMeth=Nearest
  Trip : Outport
  wires:
  C16/1 -> Arranq6/1
  Arranq6/1 -> Logical Operator4/1, Arranq6/3
  Tiempo Disparo1/1 -> Arranq6/2
  T.O./1 -> Tiempo Disparo1/2
  C15/1 -> Arranq3/1
  C14/1 -> Arranq3/3
  Arranq3/1 -> Discrete-Time Integrator/1
  Condicion arranque1/1 -> Scope1/1, Arranq3/2, Discrete-Time Integrator/2
  Pick-Up/1 -> Condicion arranque1/2
  Entrada/1 -> Condicion arranque1/1
  Discrete-Time Integrator/1 -> Scope1/2, Tiempo Disparo1/1
  Logical Operator4/1 -> Trip/1

== system HAE/Subsystem8/RMS ==
  In1 : Inport
  Absolute : MATLABFcn  MATLABFcn=abs
  Check zero Crossing : HitCross
  Constant : Constant  Value=F
  Derivative : Derivative
  Divide : Product  Inputs=/*
  Gain : Gain  Gain=2*pi
  Gain1 : Gain  Gain=1/sqrt(2)
  Hold derivative till next zero crossing : Subsystem  AncestorBlock=|  DialogController=POWERSYS.PowerSysDialog  mask(Discrete Sample & Hold){ic=0, Ts=-1}
      | powerlib_extras/Discrete 
      | Control Blocks/Discrete
      | Sample & Hold
      mask prompts: ic "Initial condition:"; Ts "Sample time:"
      mask help: The output follows input 1 (In) as long as input 2 (S) is TRUE (1) . The output is held when input 2 becomes FALSE (0). The output initial value is specified by the parameter "Initial condition".
      mask init:
      | power_initmask();
      mask Help: This block is part of a subset of blocks in the Extras library that does not have documentation associated with it, other than the block mask description.
      mask Display: disp('S/H')
  Out1 : Outport
  wires:
  Derivative/1 -> Hold derivative till next zero crossing/1(In)
  Check zero Crossing/1 -> Hold derivative till next zero crossing/2(S)
  Hold derivative till next zero crossing/1("   ") -> Absolute/1
  Constant/1 -> Gain/1
  Gain/1 -> Divide/1
  Absolute/1 -> Divide/2
  In1/1 -> Check zero Crossing/1, Derivative/1
  Divide/1 -> Gain1/1
  Gain1/1 -> Out1/1

== system HAE/Subsystem8/Timer Proteccion ==
  Entrada : Inport
  Pick-Up : Inport  Port=2
  T.O. : Inport  Port=3
  Arranq3 : Switch  Criteria=u2 ~= 0  Threshold=Ip1
  Arranq6 : Switch  Criteria=u2 ~= 0  Threshold=Ip1  ZeroCross=off
  C14 : Constant  Value=0
  C15 : Constant  Value=1000
  C16 : Constant
  Condicion arranque1 : RelationalOperator  Operator=>  OutDataTypeStr=boolean  RndMeth=Nearest
  Discrete-Time Integrator : DiscreteIntegrator  ExternalReset=falling  SampleTime=-1  ICPrevOutput=DiscIntNeverNeededParam  ICPrevScaledInput=DiscIntNeverNeededParam
  Logical Operator4 : Logic  Operator=NOT  AllPortsSameDT=off  OutDataTypeStr=boolean
  Tiempo Disparo1 : RelationalOperator  Operator=>  OutDataTypeStr=boolean  RndMeth=Nearest
  Trip : Outport
  wires:
  C16/1 -> Arranq6/1
  Arranq6/1 -> Logical Operator4/1, Arranq6/3
  Tiempo Disparo1/1 -> Arranq6/2
  T.O./1 -> Tiempo Disparo1/2
  C15/1 -> Arranq3/1
  C14/1 -> Arranq3/3
  Arranq3/1 -> Discrete-Time Integrator/1
  Condicion arranque1/1 -> Arranq3/2, Discrete-Time Integrator/2
  Pick-Up/1 -> Condicion arranque1/2
  Entrada/1 -> Condicion arranque1/1
  Discrete-Time Integrator/1 -> Tiempo Disparo1/1
  Logical Operator4/1 -> Trip/1

== system HAE/Subsystem8/Timer Proteccion1 ==
  Entrada : Inport
  Pick-Up : Inport  Port=2
  T.O. : Inport  Port=3
  Arranq3 : Switch  Criteria=u2 ~= 0  Threshold=Ip1
  Arranq6 : Switch  Criteria=u2 ~= 0  Threshold=Ip1  ZeroCross=off
  C14 : Constant  Value=0
  C15 : Constant  Value=1000
  C16 : Constant
  Condicion arranque1 : RelationalOperator  Operator=>  OutDataTypeStr=boolean  RndMeth=Nearest
  Discrete-Time Integrator : DiscreteIntegrator  ExternalReset=falling  SampleTime=-1  ICPrevOutput=DiscIntNeverNeededParam  ICPrevScaledInput=DiscIntNeverNeededParam
  Logical Operator4 : Logic  Operator=NOT  AllPortsSameDT=off  OutDataTypeStr=boolean
  Scope1 : Scope  NumInputPorts=2
  Tiempo Disparo1 : RelationalOperator  Operator=>  OutDataTypeStr=boolean  RndMeth=Nearest
  Trip : Outport
  wires:
  C16/1 -> Arranq6/1
  Arranq6/1 -> Logical Operator4/1, Arranq6/3
  Tiempo Disparo1/1 -> Arranq6/2
  T.O./1 -> Tiempo Disparo1/2
  C15/1 -> Arranq3/1
  C14/1 -> Arranq3/3
  Arranq3/1 -> Discrete-Time Integrator/1
  Condicion arranque1/1 -> Scope1/1, Arranq3/2, Discrete-Time Integrator/2
  Pick-Up/1 -> Condicion arranque1/2
  Entrada/1 -> Condicion arranque1/1
  Discrete-Time Integrator/1 -> Scope1/2, Tiempo Disparo1/1
  Logical Operator4/1 -> Trip/1
